simulink model "InvertedPendulumSystem"  (R2019a)
settings: Solver=VariableStepAuto  StartTime=0.0  StopTime=10.0  RelTol=1e-3
values from neighbouring files (symbols this model uses):
  b = 0.1    [InitializeVariables.m]
  I = 0.006    [InitializeVariables.m]
  l = 0.5    [InitializeVariables.m]
  M = 2    [InitializeVariables.m]
  m = 0.1    [InitializeVariables.m]
settings Model: Creator=jdavis6874  LastModifiedBy=jdavis6874

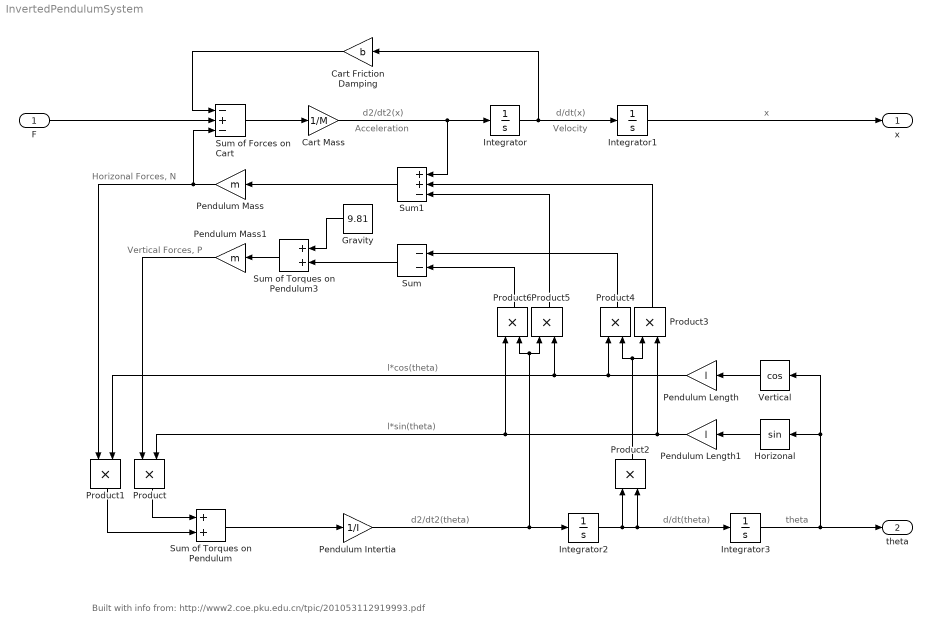
== system InvertedPendulumSystem ==
  note: Built with info from: http://www2.coe.pku.edu.cn/tpic/201053112919993.pdf
  note: theta
  note: Horizonal Forces, N
  note: l*cos(theta)
  note: d/dt(x)
  note: d2/dt2(x)
  note: d2/dt2(theta)
  note: d/dt(theta)
  note: Acceleration
  note: Velocity
  note: l*sin(theta)
  note: Vertical Forces, P
  note: x
  F : Inport
  Cart Friction Damping : Gain  Gain=b
  Cart Mass : Gain  Gain=1/M
  Gravity : Constant  Value=9.81
  Horizonal : Trigonometry
  Integrator{,1..3} (4 alike) : Integrator
  Pendulum Intertia : Gain  Gain=1/I
  Pendulum Length : Gain  Gain=l
  Pendulum Length1 : Gain  Gain=l
  Pendulum Mass : Gain  Gain=m
  Pendulum Mass1 : Gain  Gain=m
  Product{,1..6} (7 alike) : Product
  Sum : Sum  Inputs=--
  Sum of Forces on Cart : Sum  Inputs=-+-
  Sum of Torques on Pendulum : Sum
  Sum of Torques on Pendulum3 : Sum
  Sum1 : Sum  Inputs=++-
  Vertical : Trigonometry  Operator=cos
  x : Outport
  theta : Outport  Port=2
  wires:
  Sum of Forces on Cart/1 -> Cart Mass/1
  Cart Mass/1 -> Sum1/1, Integrator/1
  Integrator/1 -> Cart Friction Damping/1, Integrator1/1
  Sum of Torques on Pendulum/1 -> Pendulum Intertia/1
  F/1 -> Sum of Forces on Cart/2
  Cart Friction Damping/1 -> Sum of Forces on Cart/1
  Integrator3/1 -> theta/1, Vertical/1, Horizonal/1
  Horizonal/1 -> Pendulum Length1/1
  Vertical/1 -> Pendulum Length/1
  Integrator1/1 -> x/1
  Pendulum Length1/1 -> Product3/2, Product6/1, Product/2
  Pendulum Length/1 -> Product4/1, Product5/2, Product1/2
  Sum of Torques on Pendulum3/1 -> Pendulum Mass1/1
  Sum/1 -> Sum of Torques on Pendulum3/2
  Gravity/1 -> Sum of Torques on Pendulum3/1
  Sum1/1 -> Pendulum Mass/1
  Integrator2/1 -> Product2/1, Product2/2, Integrator3/1
  Product2/1 -> Product3/1, Product4/2
  Pendulum Intertia/1 -> Product6/2, Product5/1, Integrator2/1
  Product6/1 -> Sum/2
  Product5/1 -> Sum1/3
  Product4/1 -> Sum/1
  Product3/1 -> Sum1/2
  Pendulum Mass/1 -> Sum of Forces on Cart/3, Product1/1
  Pendulum Mass1/1 -> Product/1
  Product/1 -> Sum of Torques on Pendulum/1
  Product1/1 -> Sum of Torques on Pendulum/2
